simulink model "slex"  (Simulink 7.2)
settings: Solver=ode45  StartTime=0.0  StopTime=50  FixedStep=0.002  RelTol=1e-3
settings Model: Creator=controle  LastModifiedBy=controle  ExtModeTrigDuration=5000
settings SolverCC: PositivePriorityOrder=on
settings RTWCC: SystemTargetFile=quarc_windows.tlc  TemplateMakefile=quarc_default_tmf  Description=QUARC Win32 Target  ProcessScript=quarc_windows_make_rtw_hook
settings STFCustomTargetCC: TargetPreCompLibLocation=C:\DOCUME~1\ALLUSE~1\DADOSD~1\QUARC\lib\2008b\windows\release  SystemTargetFile=quarc_windows.tlc
settings GRTTargetCC: TargetPreCompLibLocation=C:\DOCUME~1\ALLUSE~1\DADOSD~1\QUARC\lib\2008b\windows\release  CompOptLevelCompliant=off  MatFileLogging=off  ExtMode=on  ExtModeMexFile=quarc_comm

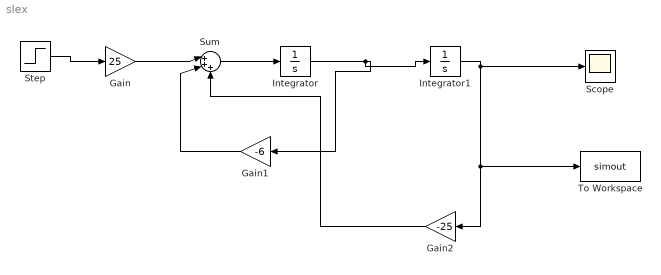
== system slex ==
  Gain : Gain  Gain=25  ParameterDataType=sfix(16)  ParameterScaling=2^0  OutDataType=sfix(16)  OutScaling=2^0
  Gain1 : Gain  Orientation=left  Gain=-6  ParameterDataType=sfix(16)  ParameterScaling=2^0  OutDataType=sfix(16)  OutScaling=2^0
  Gain2 : Gain  Orientation=left  Gain=-25  ParameterDataType=sfix(16)  ParameterScaling=2^0  OutDataType=sfix(16)  OutScaling=2^0
  Integrator : Integrator
  Integrator1 : Integrator
  Scope : Scope
      settings: TimeRange=1
  Step : Step  SampleTime=0
  Sum : Sum  Inputs=|+++  OutDataType=sfix(16)  OutScaling=2^0
  To Workspace : ToWorkspace  VariableName=simout  SampleTime=-1  SaveFormat=Structure
  wires:
  Gain/1 -> Sum/1
  Step/1 -> Gain/1
  Gain1/1 -> Sum/2
  Gain2/1 -> Sum/3
  Integrator/1 -> Gain1/1, Integrator1/1
  Integrator1/1 -> Scope/1, Gain2/1, To Workspace/1
  Sum/1 -> Integrator/1
